simulink subsystem "smc_controller"  (R2025a)
settings: Solver=VariableStepAuto  StartTime=0.0  StopTime=10.0  RelTol=1e-3
libraries: slpidlib x3, simulink_extras x2
settings Model: Creator=johnpye  LastModifiedBy=johnpye

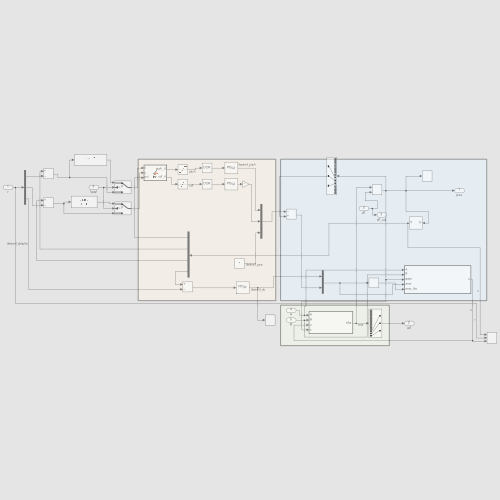
[thumbnail: Simulink's stored preview of the top-level diagram]
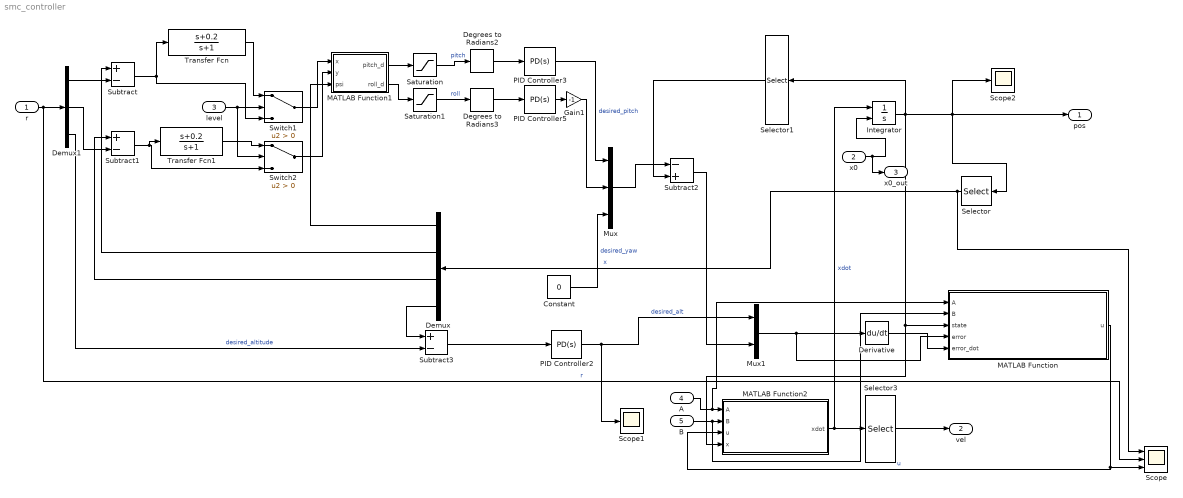
== system smc_controller ==
  r : Inport
  x0 : Inport  Port=2
  level : Inport  Port=3
  A : Inport  Port=4
  B : Inport  Port=5
  Constant : Constant  Value=0
  Degrees to Radians2 : simulink_extras/Transformations/Degrees to Radians
  Degrees to Radians3 : simulink_extras/Transformations/Degrees to Radians
  Demux : Demux
  Demux1 : Demux  Outputs=3
  Derivative : Derivative
  Gain1 : Gain  Gain=-1
  Integrator : Integrator  InitialConditionSource=external
  MATLAB Function : MATLAB Function  TreatAsAtomicUnit=on
  MATLAB Function1 : MATLAB Function  TreatAsAtomicUnit=on
  MATLAB Function2 : MATLAB Function  TreatAsAtomicUnit=on
  Mux : Mux  Inputs=3
  Mux1 : Mux  Inputs=2
  PID Controller2 : slpidlib/PID Controller  Controller=PD  Form=Parallel  TimeDomain=Continuous-time  UseExternalTs=off  SampleTime=-1  IntegratorMethod=Forward Euler  FilterMethod=Forward Euler  ControllerParametersSource=internal  P=2  I=0  UseKiTs=off  D=0  UseExternalDerivativeSource=off  N=100  UseFilter=on  TunerSelectOption=Transfer Function Based (PID Tuner App)  InitialConditionSource=internal  InitialConditionForIntegrator=0  InitialConditionForFilter=0  DifferentiatorICPrevScaledInput=0  ExternalReset=none  TrackingMode=off  Kt=1  LimitOutput=off  SatLimitsSource=internal  UpperSaturationLimit=inf  LowerSaturationLimit=-inf  LinearizeAsGain=on  AntiWindupMode=none  Kb=1  LimitIntegrator=off  UpperIntegratorSaturationLimit=inf  LowerIntegratorSaturationLimit=-inf  POutMin=[]  POutMax=[]  IOutMin=[]  IOutMax=[]  DOutMin=[]  DOutMax=[]  NOutMin=[]  NOutMax=[]  SumOutMin=[]  SumOutMax=[]  SaturationOutMin=[]  SaturationOutMax=[]  PParamMin=[]  PParamMax=[]  IParamMin=[]  IParamMax=[]  DParamMin=[]  DParamMax=[]  NParamMin=[]  NParamMax=[]  KbParamMin=[]  KbParamMax=[]  KtParamMin=[]  KtParamMax=[]  KbOutMin=[]  KbOutMax=[]  KtOutMin=[]  KtOutMax=[]  IntegratorOutMin=[]  IntegratorOutMax=[]  FilterOutMin=[]  FilterOutMax=[]  SumI1OutMin=[]  SumI1OutMax=[]  SumI2OutMin=[]  SumI2OutMax=[]  SumI3OutMin=[]  SumI3OutMax=[]  SumI4OutMin=[]  SumI4OutMax=[]  SumDOutMin=[]  SumDOutMax=[]  DifferentiatorOutMin=[]  DifferentiatorOutMax=[]  FilterDiffOutCoefMin=[]  FilterDiffOutCoefMax=[]  ReciprocalOutMin=[]  ReciprocalOutMax=[]  SumDenOutMin=[]  SumDenOutMax=[]  SumNumOutMin=[]  SumNumOutMax=[]  DivideOutMin=[]  DivideOutMax=[]  UdiffTsProdOutMin=[]  UdiffTsProdOutMax=[]  NTsProdOutMin=[]  NTsProdOutMax=[]  UintegralTsProdOutMin=[]  UintegralTsProdOutMax=[]  UngainTsProdOutMin=[]  UngainTsProdOutMax=[]  ClampingZeroOutDataTypeStr=Inherit: Inherit via back propagation  ClampingZeroOutMin=[]  ClampingZeroOutMax=[]  FilterDenConstantOutDataTypeStr=Inherit: Inherit via back propagation  FilterDenConstantOutMin=[]  FilterDenConstantOutMax=[]  PCopyOutDataTypeStr=Inherit: Inherit via back propagation  PCopyOutMin=[]  PCopyOutMax=[]  NCopyOutDataTypeStr=Inherit: Inherit via back propagation  NCopyOutMin=[]  NCopyOutMax=[]  IntegratorContinuousStateAttributes=''  IntegratorStateMustResolveToSignalObject=off  IntegratorRTWStateStorageClass=Auto  FilterContinuousStateAttributes=''  FilterStateMustResolveToSignalObject=off  FilterRTWStateStorageClass=Auto  ParallelPVariant=InternalParameters  IdealPVariant=Disabled  IVariant=Disabled  DVariant=InternalParameters  IntegratorVariant=Disabled  SatVariant=Disabled  AWVariant=Disabled  PCopyVariant=Disabled  TRVariant=Disabled  FdbkBlocksVariant=Forward  IdealPFdbkVariant=Disabled  SatFdbkVariant=Disabled  DerivativeFilterVariant=ContFilter  NVariant=InternalParameters  NCopyVariant=Disabled  FilterICVariant=InternalICsFilter  IntegratorICVariant=Disabled  ExternalResetVariant=Disabled  TRSumVariant=Passthrough  SumFdbkVariant=Disabled  SumVariant=Sum_PD  TsampFilterVariant=InternalTs  TsampNgainVariant=Passthrough  TsampIntegralVariant=Disabled_SignalSpec  ExternalSaturationOutDataTypeStr=Inherit: Same as second input  DerivativeSourceVariant=ErrorSignal  PreIntVariant=InternalPreInt
  PID Controller3 : slpidlib/PID Controller  Controller=PD  Form=Parallel  TimeDomain=Continuous-time  UseExternalTs=off  SampleTime=-1  IntegratorMethod=Forward Euler  FilterMethod=Forward Euler  ControllerParametersSource=internal  P=4  I=0  UseKiTs=off  D=10  UseExternalDerivativeSource=off  N=50  UseFilter=on  TunerSelectOption=Transfer Function Based (PID Tuner App)  InitialConditionSource=internal  InitialConditionForIntegrator=0  InitialConditionForFilter=0  DifferentiatorICPrevScaledInput=0  ExternalReset=none  TrackingMode=off  Kt=1  LimitOutput=off  SatLimitsSource=internal  UpperSaturationLimit=inf  LowerSaturationLimit=-inf  LinearizeAsGain=on  AntiWindupMode=none  Kb=1  LimitIntegrator=off  UpperIntegratorSaturationLimit=inf  LowerIntegratorSaturationLimit=-inf  POutMin=[]  POutMax=[]  IOutMin=[]  IOutMax=[]  DOutMin=[]  DOutMax=[]  NOutMin=[]  NOutMax=[]  SumOutMin=[]  SumOutMax=[]  SaturationOutMin=[]  SaturationOutMax=[]  PParamMin=[]  PParamMax=[]  IParamMin=[]  IParamMax=[]  DParamMin=[]  DParamMax=[]  NParamMin=[]  NParamMax=[]  KbParamMin=[]  KbParamMax=[]  KtParamMin=[]  KtParamMax=[]  KbOutMin=[]  KbOutMax=[]  KtOutMin=[]  KtOutMax=[]  IntegratorOutMin=[]  IntegratorOutMax=[]  FilterOutMin=[]  FilterOutMax=[]  SumI1OutMin=[]  SumI1OutMax=[]  SumI2OutMin=[]  SumI2OutMax=[]  SumI3OutMin=[]  SumI3OutMax=[]  SumI4OutMin=[]  SumI4OutMax=[]  SumDOutMin=[]  SumDOutMax=[]  DifferentiatorOutMin=[]  DifferentiatorOutMax=[]  FilterDiffOutCoefMin=[]  FilterDiffOutCoefMax=[]  ReciprocalOutMin=[]  ReciprocalOutMax=[]  SumDenOutMin=[]  SumDenOutMax=[]  SumNumOutMin=[]  SumNumOutMax=[]  DivideOutMin=[]  DivideOutMax=[]  UdiffTsProdOutMin=[]  UdiffTsProdOutMax=[]  NTsProdOutMin=[]  NTsProdOutMax=[]  UintegralTsProdOutMin=[]  UintegralTsProdOutMax=[]  UngainTsProdOutMin=[]  UngainTsProdOutMax=[]  ClampingZeroOutDataTypeStr=Inherit: Inherit via back propagation  ClampingZeroOutMin=[]  ClampingZeroOutMax=[]  FilterDenConstantOutDataTypeStr=Inherit: Inherit via back propagation  FilterDenConstantOutMin=[]  FilterDenConstantOutMax=[]  PCopyOutDataTypeStr=Inherit: Inherit via back propagation  PCopyOutMin=[]  PCopyOutMax=[]  NCopyOutDataTypeStr=Inherit: Inherit via back propagation  NCopyOutMin=[]  NCopyOutMax=[]  IntegratorContinuousStateAttributes=''  IntegratorStateMustResolveToSignalObject=off  IntegratorRTWStateStorageClass=Auto  FilterContinuousStateAttributes=''  FilterStateMustResolveToSignalObject=off  FilterRTWStateStorageClass=Auto  ParallelPVariant=InternalParameters  IdealPVariant=Disabled  IVariant=Disabled  DVariant=InternalParameters  IntegratorVariant=Disabled  SatVariant=Disabled  AWVariant=Disabled  PCopyVariant=Disabled  TRVariant=Disabled  FdbkBlocksVariant=Forward  IdealPFdbkVariant=Disabled  SatFdbkVariant=Disabled  DerivativeFilterVariant=ContFilter  NVariant=InternalParameters  NCopyVariant=Disabled  FilterICVariant=InternalICsFilter  IntegratorICVariant=Disabled  ExternalResetVariant=Disabled  TRSumVariant=Passthrough  SumFdbkVariant=Disabled  SumVariant=Sum_PD  TsampFilterVariant=InternalTs  TsampNgainVariant=Passthrough  TsampIntegralVariant=Disabled_SignalSpec  ExternalSaturationOutDataTypeStr=Inherit: Same as second input  DerivativeSourceVariant=ErrorSignal  PreIntVariant=InternalPreInt
  PID Controller5 : slpidlib/PID Controller  Controller=PD  Form=Parallel  TimeDomain=Continuous-time  UseExternalTs=off  SampleTime=-1  IntegratorMethod=Forward Euler  FilterMethod=Forward Euler  ControllerParametersSource=internal  P=4  I=0  UseKiTs=off  D=10  UseExternalDerivativeSource=off  N=50  UseFilter=on  TunerSelectOption=Transfer Function Based (PID Tuner App)  InitialConditionSource=internal  InitialConditionForIntegrator=0  InitialConditionForFilter=0  DifferentiatorICPrevScaledInput=0  ExternalReset=none  TrackingMode=off  Kt=1  LimitOutput=off  SatLimitsSource=internal  UpperSaturationLimit=inf  LowerSaturationLimit=-inf  LinearizeAsGain=on  AntiWindupMode=none  Kb=1  LimitIntegrator=off  UpperIntegratorSaturationLimit=inf  LowerIntegratorSaturationLimit=-inf  POutMin=[]  POutMax=[]  IOutMin=[]  IOutMax=[]  DOutMin=[]  DOutMax=[]  NOutMin=[]  NOutMax=[]  SumOutMin=[]  SumOutMax=[]  SaturationOutMin=[]  SaturationOutMax=[]  PParamMin=[]  PParamMax=[]  IParamMin=[]  IParamMax=[]  DParamMin=[]  DParamMax=[]  NParamMin=[]  NParamMax=[]  KbParamMin=[]  KbParamMax=[]  KtParamMin=[]  KtParamMax=[]  KbOutMin=[]  KbOutMax=[]  KtOutMin=[]  KtOutMax=[]  IntegratorOutMin=[]  IntegratorOutMax=[]  FilterOutMin=[]  FilterOutMax=[]  SumI1OutMin=[]  SumI1OutMax=[]  SumI2OutMin=[]  SumI2OutMax=[]  SumI3OutMin=[]  SumI3OutMax=[]  SumI4OutMin=[]  SumI4OutMax=[]  SumDOutMin=[]  SumDOutMax=[]  DifferentiatorOutMin=[]  DifferentiatorOutMax=[]  FilterDiffOutCoefMin=[]  FilterDiffOutCoefMax=[]  ReciprocalOutMin=[]  ReciprocalOutMax=[]  SumDenOutMin=[]  SumDenOutMax=[]  SumNumOutMin=[]  SumNumOutMax=[]  DivideOutMin=[]  DivideOutMax=[]  UdiffTsProdOutMin=[]  UdiffTsProdOutMax=[]  NTsProdOutMin=[]  NTsProdOutMax=[]  UintegralTsProdOutMin=[]  UintegralTsProdOutMax=[]  UngainTsProdOutMin=[]  UngainTsProdOutMax=[]  ClampingZeroOutDataTypeStr=Inherit: Inherit via back propagation  ClampingZeroOutMin=[]  ClampingZeroOutMax=[]  FilterDenConstantOutDataTypeStr=Inherit: Inherit via back propagation  FilterDenConstantOutMin=[]  FilterDenConstantOutMax=[]  PCopyOutDataTypeStr=Inherit: Inherit via back propagation  PCopyOutMin=[]  PCopyOutMax=[]  NCopyOutDataTypeStr=Inherit: Inherit via back propagation  NCopyOutMin=[]  NCopyOutMax=[]  IntegratorContinuousStateAttributes=''  IntegratorStateMustResolveToSignalObject=off  IntegratorRTWStateStorageClass=Auto  FilterContinuousStateAttributes=''  FilterStateMustResolveToSignalObject=off  FilterRTWStateStorageClass=Auto  ParallelPVariant=InternalParameters  IdealPVariant=Disabled  IVariant=Disabled  DVariant=InternalParameters  IntegratorVariant=Disabled  SatVariant=Disabled  AWVariant=Disabled  PCopyVariant=Disabled  TRVariant=Disabled  FdbkBlocksVariant=Forward  IdealPFdbkVariant=Disabled  SatFdbkVariant=Disabled  DerivativeFilterVariant=ContFilter  NVariant=InternalParameters  NCopyVariant=Disabled  FilterICVariant=InternalICsFilter  IntegratorICVariant=Disabled  ExternalResetVariant=Disabled  TRSumVariant=Passthrough  SumFdbkVariant=Disabled  SumVariant=Sum_PD  TsampFilterVariant=InternalTs  TsampNgainVariant=Passthrough  TsampIntegralVariant=Disabled_SignalSpec  ExternalSaturationOutDataTypeStr=Inherit: Same as second input  DerivativeSourceVariant=ErrorSignal  PreIntVariant=InternalPreInt
  Saturation : Saturate  UpperLimit=30  LowerLimit=-30
  Saturation1 : Saturate  UpperLimit=30  LowerLimit=-30
  Scope : Scope  NumInputPorts=3
      settings: ActiveDisplayYMinimum=-2.4108987743999928E+16  ActiveDisplayYMaximum=7.4768819203398432E+16  DataLoggingVariableName=ScopeData19
  Scope1 : Scope
      settings: ActiveDisplayYMinimum=324.95318009295426  ActiveDisplayYMaximum=724.47010254885754  DataLoggingVariableName=ScopeData20
  Scope2 : Scope
      settings: ActiveDisplayYMinimum=-7.7734913190096284  ActiveDisplayYMaximum=11.974832368778847
  Selector : Selector  InputPortWidth=12  IndexOptions=Index vector (dialog)  Indices=[9 10 11 12]  OutputSizes=1
  Selector1 : Selector  InputPortWidth=12  IndexOptions=Index vector (dialog)  Indices=[7 8 9]  OutputSizes=1
  Selector3 : Selector  InputPortWidth=12  IndexOptions=Index vector (dialog)  Indices=[10 11 12]  OutputSizes=1
  Subtract : Sum  Inputs=+-
  Subtract1 : Sum  Inputs=+-
  Subtract2 : Sum  Inputs=-+
  Subtract3 : Sum  Inputs=+-
  Switch1 : Switch  Criteria=u2 > Threshold  SaturateOnIntegerOverflow=off  InputSameDT=off
  Switch2 : Switch  Criteria=u2 > Threshold  SaturateOnIntegerOverflow=off  InputSameDT=off
  Transfer Fcn : TransferFcn  Numerator=[1 0.2]  Denominator=[1 1]
  Transfer Fcn1 : TransferFcn  Numerator=[1 0.2]  Denominator=[1 1]
  pos : Outport
  vel : Outport  Port=2
  x0_out : Outport  Port=3
  wires:
  Selector3/1 -> vel/1
  Mux1/1 -> MATLAB Function/4(error), Derivative/1
  x0/1 -> Integrator/2, x0_out/1
  Selector1/1 -> Subtract2/2
  A/1 -> MATLAB Function2/1(A), MATLAB Function/1(A)
  Mux/1 -> Subtract2/1
  Subtract/1 -> Transfer Fcn/1, Switch1/3
  Switch2/1 -> MATLAB Function1/2(y)
  Subtract2/1 -> Mux1/2
  Demux/1 -> MATLAB Function1/3(psi)
  Subtract3/1 -> PID Controller2/1
  Integrator/1 -> Selector1/1, pos/1, Scope2/1, Selector/1, MATLAB Function/3(state), MATLAB Function2/4(x)
  Demux/3 -> Subtract1/1
  B/1 -> MATLAB Function2/2(B), MATLAB Function/2(B)
  Demux1/2 -> Subtract1/2
  level/1 -> Switch1/2, Switch2/2
  MATLAB Function2/1(xdot) -> Integrator/1, Selector3/1  "xdot"
  PID Controller2/1 -> Mux1/1, Scope1/1  "desired_alt"
  Transfer Fcn/1 -> Switch1/1
  Derivative/1 -> MATLAB Function/5(error_dot)
  Switch1/1 -> MATLAB Function1/1(x)
  r/1 -> Demux1/1, Scope/2  "r"
  MATLAB Function/1(u) -> Scope/3, MATLAB Function2/3(u)  "u"
  Constant/1 -> Mux/3  "desired_yaw"
  Transfer Fcn1/1 -> Switch2/1
  Demux/2 -> Subtract/1
  Demux1/1 -> Subtract/2
  Subtract1/1 -> Transfer Fcn1/1, Switch2/3
  Selector/1 -> Demux/1, Scope/1  "x"
  Demux/4 -> Subtract3/1
  Demux1/3 -> Subtract3/2  "desired_altitude"
  MATLAB Function1/1(pitch_d) -> Saturation/1
  Saturation/1 -> Degrees to Radians2/1  "pitch"
  Saturation1/1 -> Degrees to Radians3/1  "roll"
  MATLAB Function1/2(roll_d) -> Saturation1/1
  Degrees to Radians2/1 -> PID Controller3/1
  Degrees to Radians3/1 -> PID Controller5/1
  PID Controller5/1 -> Gain1/1
  PID Controller3/1 -> Mux/1  "desired_pitch"
  Gain1/1 -> Mux/2

== matlab function smc_controller/MATLAB Function ==
  data: A input; B input; state input; u output; error input; error_dot input
function u = smc_attitude(A,B,state, error, error_dot)

g = 9.81; % m/s^2
l = 0.2; % m
m = 0.8; % kg
Jmp = 0;
Jxx = 1.8e-3; % kgm^2
Jyy = 1.8e-3; % kgm^2
Jzz = 1.5e-3; % kgm^2
kmt = 0.1; % m

% K = B(4,2)*Jxx;
% m = (1/B(3,1)) * -K;

u = zeros(4,1);

vx = state(1);
vy = state(2);
vz = state(3);
wx = state(4);
wy = state(5);
wz = state(6);

theta = state(7);
phi = state(8);
psi = state(9);
z = state(12);

eT = error(1);
eTheta = error(2);
ePhi = error(3);
ePsi = error(4);

eT_dot = error_dot(1);
eTheta_dot = error_dot(2);
ePhi_dot = error_dot(3);
ePsi_dot = error_dot(4);

KT = 12*m/(cos(theta)*cos(phi)); % this term is basically thrust response
KMx = 8*Jxx;
KMy = 8*Jyy/cos(phi);
KMz = Jzz*cos(theta)/cos(phi);

beta = 0.5;

cT = 6;
cX = 10;
cY = 10;
cZ = 0.5;

sT = cT*eT + eT_dot; % noto bene, this is not a feedback formulation
sT = min([sT/beta 1]);
sT = max([sT/beta -1]);

sMx = cX*ePhi + ePhi_dot;
sMx = min([sMx/beta 1]);
sMx = max([sMx/beta -1]);

sMy = cY*eTheta + eTheta_dot;
sMy = min([sMy/beta 1]);
sMy = max([sMy/beta -1]);

sMz = cZ*ePsi + ePsi_dot;
sMz = min([sMz/beta 1]);
sMz = max([sMz/beta -1]);

uhat_T = (-m*cT/(cos(theta)*cos(phi)))*(vx*sin(theta) - vy*cos(theta)*sin(phi) - vz*cos(theta)*cos(phi)) + m*(-vy*wx + vx*wy + g*cos(theta)*cos(phi));
uhat_Mx = -cX*Jxx*(wx + wy*sin(phi)*tan(theta) + wz*cos(phi)*tan(theta)) + wy*wz*(Jzz-Jyy);
uhat_My = (-cY*Jzz/cos(phi))*(wy*cos(phi) - wz*sin(phi)) + wx*wz*(Jxx-Jzz);
uhat_Mz = -cZ*Jzz*(wy*tan(phi) + wz);

u_T = uhat_T - KT*sT;
u_Mx = uhat_Mx - KMx*sMx;
u_My = uhat_My - KMy*sMy;
u_Mz = uhat_Mz - KMz*sMz;

u(1) = u_T;
u(2) = u_Mx;
u(3) = u_My;
u(4) = u_Mz;

== matlab function smc_controller/MATLAB Function1 ==
  data: pitch_d output; x input; y input; psi input; roll_d output
function [pitch_d, roll_d] = fcn(x, y, psi)

R = [cos(psi) -sin(psi); sin(psi) cos(psi)];
res = R*[x; y];
pitch_d = res(1);
roll_d = res(2);

== matlab function smc_controller/MATLAB Function2 ==
  data: A input; B input; u input; x input; xdot output
function xdot = system_dynamics(A, B, u, x)

g = 9.81; % m/s^2
l = 0.2; % m
Jmp = 0;
Jxx = 1.8e-3; % kgm^2
Jyy = 1.8e-3; % kgm^2
Jzz = 1.5e-3; % kgm^2
kmt = 0.1; % m

K = B(4,2)*Jxx;
m = (1/B(3,1)) * -K;

u = reshape(u, [4, 1]);
x = reshape(x, [12, 1]);
% xdot = A*x + B*u;
xdot=zeros(12,1);

vx = x(1);
vy = x(2);
vz = x(3);
wx = x(4);
wy = x(5);
wz = x(6);
theta = x(7);
phi = x(8);
psi = x(9);
% T = K*u(1);
% Mx = K*u(2);
% My = K*u(3);
% Mz = K*u(4);
T = u(1);
Mx = u(2);
My = u(3);
Mz = u(4);

% Step 3: Calculate derivatives
xdot(1)         = -vz*wy + vy*wz - g*sin(theta);
xdot(2)         = -vx*wz + vz*wx + g*cos(theta)*sin(phi);
xdot(3)         = -vy*wx + vx*wy + g*cos(theta)*cos(phi) - T/m;
xdot(4)         = (1/Jxx)*(-wy*wz*(Jzz - Jyy) + Mx);
xdot(5)         = (1/Jyy)*(-wx*wz*(Jxx - Jzz) + My);
xdot(6)         = Mz / Jzz;
xdot(7)         = wy*cos(phi) - wz*sin(phi);
xdot(8)         = wx + wy*sin(phi)*tan(theta) + wz*cos(phi)*tan(theta);
xdot(9)         = wy*(sin(phi)/cos(theta)) + wz*(cos(phi)/cos(theta));
xdot(10)        = vx*cos(psi)*cos(theta) + ...
                    vy*(-sin(psi)*cos(phi) + cos(psi)*sin(theta)*sin(phi)) + ...
                    vz*(sin(psi)*sin(phi) + cos(psi)*sin(theta)*cos(phi));
xdot(11)        = vx*sin(psi)*cos(theta) + ...
                    vy*(cos(psi)*cos(phi) + sin(psi)*sin(theta)*sin(phi)) + ...
                    vz*(-cos(psi)*sin(phi) + sin(psi)*sin(theta)*cos(phi));
xdot(12)        = vx*sin(theta) - vy*cos(theta)*sin(phi) - vz*cos(theta)*cos(phi);
